simulink model "DSSS_Final"  (R2020a)
settings: Solver=VariableStepAuto  StartTime=0.0  StopTime=10.0  RelTol=1e-3
libraries: commutil2 x2, msbUtilities x1, dspfdesign x1, commseqgen3 x1, dspsrcs4 x1, simulink x1
settings Model: Creator=Diganta  LastModifiedBy=Diganta
settings DebuggingCC: SFMachineParentedDataDiag=error

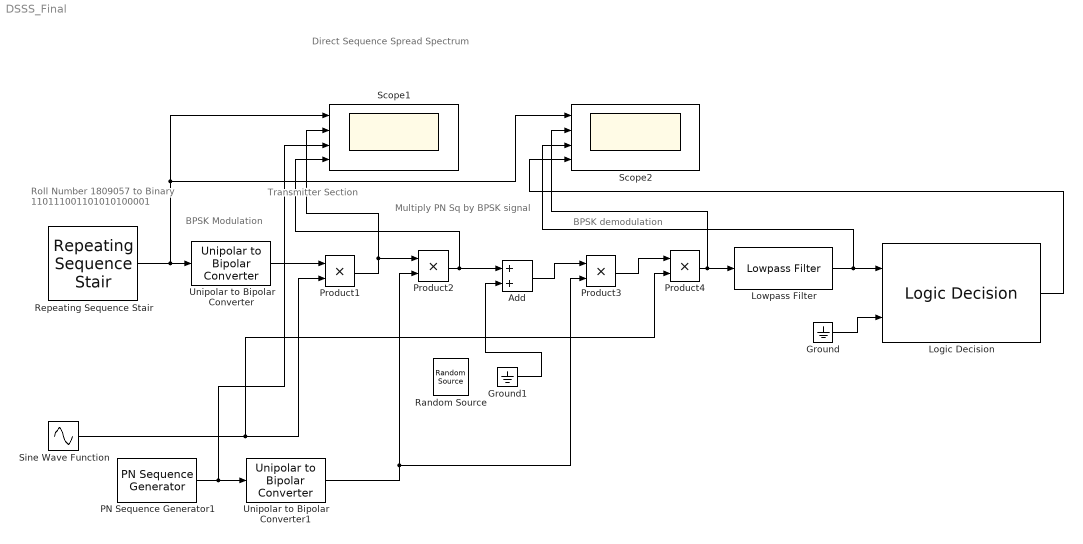
== system DSSS_Final ==
  note: Direct Sequence Spread Spectrum
  note: BPSK demodulation
  note: Transmitter Section
  note: Multiply PN Sq
      | by BPSK signal
  note: BPSK Modulation
  note: Roll Number 1809057
      | to Binary
      | 110111001101010100001
  Add : Sum
  Ground : Ground
  Ground1 : Ground
  Logic Decision : msbUtilities/Logic Decision  SampleTimeSource=Inherited  SampleTimeIn=20e-12  Delay=1e-15  BufferSizeIn=1
      settings: SourceProductBaseCode=AM
  Lowpass Filter : dspfdesign/Lowpass Filter  FilterType=IIR  DesignForMinimumOrder=off  FilterOrder=8  PassbandFrequency=50  StopbandFrequency=12e3  PassbandRipple=0.1  StopbandAttenuation=120  InheritSampleRate=off  SampleRate=44100  SimulateUsing=Interpreted execution  roundingMode=Floor  coeffsDataTypeStr=fixdt(1,16)
  PN Sequence Generator1 : commseqgen3/PN Sequence Generator  poly='z^8+z^6+z^3 + z + 1'  ini_sta=[0 1 0 1 0 1 0 0]  outBitMaskSource=Dialog parameter  shift=0  outVarSiz=off  maxOutSizeMode=Dialog parameter  maxOutSize=[10 1]  Ts=0.00001  sampPerFrame=1  reset=off  bitPackedOutputs=off  outDataType=boolean  numPackedBits=8  bitPackDataSigned=off  bitPackedOutDType=double
  Product{1..4} (4 alike) : Product
  Random Source : dspsrcs4/Random Source  SrcType=Gaussian  NormMethod=Ziggurat  CltLength=12  MinVal=1  MaxVal=1  MeanVal=1  VarVal=10  RepMode=Not repeatable  rawSeed=1  IsInherit=off  SampMode=Discrete  SampTime=1  SampFrame=1  DataType=Double  OutComplex=Real  OutputFrames=off
  Repeating Sequence Stair : simulink/Sources/Repeating Sequence Stair  OutValues=[1 1 0 1 1 1 0 0 1 1 0 1 0 1 0 1 0 0 0 0 1].'  tsamp=0.5  OutMin=[]  OutMax=[]  OutDataTypeStr=fixdt('boolean')  OutputDataTypeScalingMode=Specify via dialog  OutDataType=fixdt('boolean')  ConRadixGroup=Best Precision: Vector-wise  OutScaling=[]
  Scope1 : Scope  NumInputPorts=4
  Scope2 : Scope  NumInputPorts=4
  Sine Wave Function : Sin  Frequency=2*pi*100  Samples=10000  SampleTime=.001
  Unipolar to Bipolar Converter : commutil2/Unipolar to Bipolar Converter  M=2  polarity=Positive  dataType=double
  Unipolar to Bipolar Converter1 : commutil2/Unipolar to Bipolar Converter  M=2  polarity=Positive  dataType=double
  wires:
  Repeating Sequence Stair/1 -> Unipolar to Bipolar Converter/1, Scope2/1, Scope1/1
  Product1/1 -> Product2/1, Scope1/2
  Unipolar to Bipolar Converter/1 -> Product1/1
  Sine Wave Function/1 -> Product4/2, Product1/2
  Product2/1 -> Scope1/4, Add/1
  PN Sequence Generator1/1 -> Scope1/3, Unipolar to Bipolar Converter1/1
  Unipolar to Bipolar Converter1/1 -> Product3/2, Product2/2
  Add/1 -> Product3/1
  Product3/1 -> Product4/1
  Product4/1 -> Scope2/2, Lowpass Filter/1
  Lowpass Filter/1 -> Logic Decision/1, Scope2/3
  Ground/1 -> Logic Decision/2
  Logic Decision/1 -> Scope2/4
  Ground1/1 -> Add/2
